simulink model "Rotor_and_Motor"  (R2022b)
settings: Solver=VariableStepAuto  StartTime=0.0  StopTime=20  MaxStep=.0001  RelTol=1e-3
InitFcn:
  | dir = pwd; %model directory
  | 
  | %go to look up tables
  | cd('..\Look Up Tables') %look up table directory
  | 
  | %Ct, Cp, and theta of rotor
  | load("Look Up Tables\BEMTdata_coax_final.mat");
  | 
  | %Peters-He model parameters (M,L,shape)
  | load("Look Up Tables\PetersHe_1state.mat");
  | 
  | %go back to model directory
  | cd(pwd);
  | 
  | %Ct, Cp, and theta of rotor
  | load("Look Up Tables\BEMTdata_coax_final.mat");
  | 
  | %Peters-He model parameters (M,L,shape)
  | load("Look Up Tables\PetersHe_1state.mat");
  | 
  | %rotor parameters
  | d_prop = 2*1.016;
  | R_c = d_prop/2*.12;
  | Nb = 2;
  | dr = rotor_params.dr;
  | Inertia = rotor_params.I_rotor;
  | kappa = rotor_params.kappa;
  | Cp0 = 5.908e-5;
  | 
  | %atmospheric properties
  | rho_air = 1.225;
  | 
  | 
  | %transmission properties
  | GR = 1.2;
  | wn = 101.0346; %transmission natural freq (rad/s)
  | zeta = 0.0106; %transmission damping ratio (-)
  | % wn = 30; %transmission natural freq (rad/s)
  | % zeta = 2*0.0106; %transmission damping ratio (-)
  | K = wn^2*Inertia; %belt stiffness
  | b = 2*zeta*sqrt(Inertia*K);%0.7706; %belt damping
  | % b = 1;
  | 
  | %model conditions
  | RPM0 = 945*GR;
  | RPMf = 975*GR;
  | ramp = 200*GR; %[rpm/s]
  | k = 0.865; %mass flow correction
  | shape = model.psi_a(1);
values from neighbouring files (symbols this model uses):
  Cp = [0.000195201118563 0.000195344815163 0.000195970524669 0.000196911243155 0.000198292722473 0.000199793715635 0.000201836164013 0.000204359459521 0.00020706119236 0.00020992934584 0.000212955219574 0.000216131124695 ... (150 elements, 1x150)]    [BEMT-1.mat]    (also in BEMT-2.mat = [5.908e-05 5.908e-05 5.908e-05 5.908e-05 5.908e-05 5.908e-05; BEMT-3.mat = [6.167e-05 6.167e-05 6.167e-05 6.167e-05 6.167e-05 6.1671725; BEMT-PF-Isolated-1.mat = [6.88284627296e-05 6.76929537705e-05 6.92283244838e-05 7.518; BEMT-PF-Isolated-2.mat = [6.88286203447e-05 6.76929720507e-05 6.92293837373e-05 7.518)
  Ct = [0 8.42066058624e-05 0.000168413211725 0.000252619817587 0.000348569118235 0.000435711397794 0.000522853677352 0.000609995956911 0.00069713823647 0.000784280516029 0.000871422795587 0.000958565075146 ... (150 elements, 1x150)]    [BEMT-1.mat]    (also in BEMT-2.mat = [-0.000241284312952 -0.00019885713846 -0.000156429963968 -0.; BEMT-3.mat = [-0.000252881464423 -0.00020500571035 -0.00015767832519 -0.0; BEMT-PF-Isolated-1.mat = [-0.000124730397385 6.78902114512e-07 0.000152796242494 0.00; BEMT-PF-Isolated-2.mat = [-0.000124743531158 6.68801957239e-07 0.000152879013625 0.00)
  model =     [DynInflow-1.mat]    (also in PP-1.mat; PP-2.mat; PP-3.mat)
  rotor_params =     [DynInflow-1.mat]    (also in PP-1.mat; PP-2.mat; PP-3.mat)
  theta = [-1.24244156171 -0.730247869575 -0.489791195362 -0.291308360013 -0.0904887039498 0.0775201787218 0.236938510902 0.389966557012 0.537998944025 0.680941129328 0.820002111662 0.955737387113 ... (150 elements, 1x150)]    [BEMT-1.mat]    (also in BEMT-2.mat = [-2.67472972391 -2.52181622329 -2.35655527709 -2.17339529035; BEMT-3.mat = [-2.61565298703 -2.45920727031 -2.29202818901 -2.11251263407; BEMT-PF-Isolated-1.mat = [-2 -1 0 1 2 3 4 5 6 7 8 9 ... (16 elements, 1x16)]; BEMT-PF-Isolated-2.mat = [-2 -1 0 1 2 3 4 5 6 7 8 9 ... (16 elements, 1x16)])
libraries: simulink x1
settings Model: PacingRate=0.010000  Creator=msa2925  LastModifiedBy=asper101

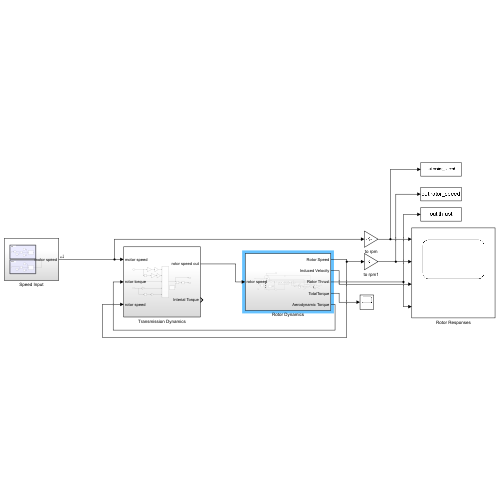
[thumbnail: Simulink's stored preview of the top-level diagram]
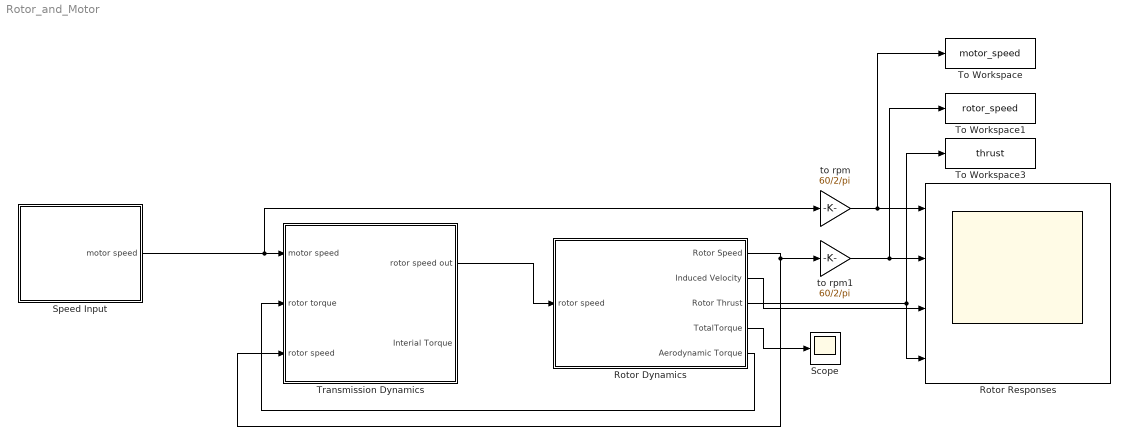
== system Rotor_and_Motor ==
  Rotor Dynamics : Subsystem
  Rotor Responses : Scope  NumInputPorts=4
  Scope : Scope
  Speed Input : Subsystem
  To Workspace : ToWorkspace  VariableName=motor_speed  SaveFormat=Timeseries  SampleTime=-1
  To Workspace1 : ToWorkspace  VariableName=rotor_speed  SaveFormat=Timeseries  SampleTime=-1
  To Workspace3 : ToWorkspace  VariableName=thrust  SaveFormat=Timeseries  SampleTime=-1
  Transmission Dynamics : Subsystem
  to rpm : Gain  Gain=60/2/pi
  to rpm1 : Gain  Gain=60/2/pi
  wires:
  Rotor Dynamics/1(Rotor Speed) -> Transmission Dynamics/3(rotor speed), to rpm1/1
  Rotor Dynamics/2(Induced Velocity) -> Rotor Responses/3
  Rotor Dynamics/3(Rotor Thrust) -> Rotor Responses/4, To Workspace3/1
  Rotor Dynamics/5(Aerodynamic Torque) -> Transmission Dynamics/2(rotor torque)
  Speed Input/1(motor speed) -> to rpm/1, Transmission Dynamics/1(motor speed)
  to rpm1/1 -> To Workspace1/1, Rotor Responses/2
  to rpm/1 -> To Workspace/1, Rotor Responses/1
  Rotor Dynamics/4(TotalTorque) -> Scope/1
  Transmission Dynamics/1(rotor speed out) -> Rotor Dynamics/1(rotor speed)

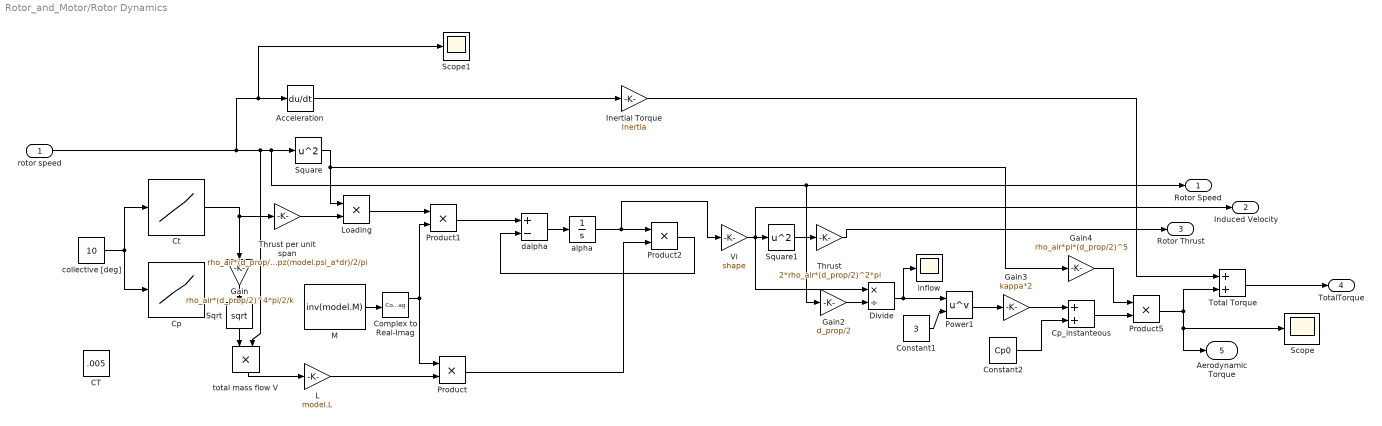
== system Rotor_and_Motor/Rotor Dynamics ==
  rotor speed : Inport
  Acceleration : Derivative
  CT : Constant  Value=.005
  Complex to Real-Imag : ComplexToRealImag
  Constant1 : Constant  Value=3
  Constant2 : Constant  Value=Cp0
  Cp : Lookup_n-D  NumberOfTableDimensions=1  BreakpointsForDimension1=theta  BreakpointsForDimension2=[1:3]  Table=Cp  InternalRulePriority=Speed  RndMeth=Simplest
  Cp_instanteous : Sum
  Ct : Lookup_n-D  NumberOfTableDimensions=1  BreakpointsForDimension1=theta  BreakpointsForDimension2=[1:3]  Table=Ct  InternalRulePriority=Speed  RndMeth=Simplest
  Divide : Product  Inputs=*/
  Gain : Gain  Gain=rho_air*(d_prop/2)^4*pi/2/k
  Gain2 : Gain  Gain=d_prop/2
  Gain3 : Gain  Gain=kappa*2
  Gain4 : Gain  Gain=rho_air*pi*(d_prop/2)^5
  Inertial Torque : Gain  Gain=Inertia
  L : Gain  Gain=model.L
  Loading : Product
  M : Constant  Value=inv(model.M)
  Power1 : Math  Operator=pow
  Product{,1..2,5} (4 alike) : Product
  Scope : Scope
  Scope1 : Scope
  Sqrt : Sqrt
  Square : Math  Operator=square
  Square1 : Math  Operator=square
  Thrust : Gain  Gain=2*rho_air*(d_prop/2)^2*pi
  Thrust per unit span : Gain  Gain=rho_air*(d_prop/2)^4*pi/(d_prop/2)*trapz(model.psi_a*dr)/2/pi
  Total Torque : Sum
  Vi : Gain  Gain=shape
  alpha : Integrator
  collective [deg] : Constant  Value=10
  dalpha : Sum  Inputs=+-
  inflow : Scope
  total mass flow V : Product
  Rotor Speed : Outport
  Induced Velocity : Outport  Port=2
  Rotor Thrust : Outport  Port=3
  TotalTorque : Outport  Port=4
  Aerodynamic Torque : Outport  Port=5
  wires:
  Gain/1 -> Sqrt/1
  L/1 -> Product/2
  total mass flow V/1 -> L/1
  collective [deg]/1 -> Cp/1, Ct/1
  Product2/1 -> dalpha/2
  rotor speed/1 -> Scope1/1, Acceleration/1, Square/1, Rotor Speed/1, Gain2/1, total mass flow V/2
  Vi/1 -> Induced Velocity/1, Divide/1, Square1/1
  Sqrt/1 -> total mass flow V/1
  Loading/1 -> Product1/1
  Product/1 -> Product2/2
  Square1/1 -> Thrust/1
  dalpha/1 -> alpha/1
  Thrust/1 -> Rotor Thrust/1
  Ct/1 -> Thrust per unit span/1, Gain/1
  M/1 -> Complex to Real-Imag/1
  Product1/1 -> dalpha/1
  alpha/1 -> Vi/1, Product2/1
  Complex to Real-Imag/1 -> Product1/2, Product/1
  Thrust per unit span/1 -> Loading/2
  Total Torque/1 -> TotalTorque/1
  Inertial Torque/1 -> Total Torque/1
  Acceleration/1 -> Inertial Torque/1
  Gain2/1 -> Divide/2
  Power1/1 -> Gain3/1
  Gain3/1 -> Cp_instanteous/1
  Constant2/1 -> Cp_instanteous/2
  Square/1 -> Loading/1, Gain4/1
  Gain4/1 -> Product5/1
  Cp_instanteous/1 -> Product5/2
  Constant1/1 -> Power1/2
  Divide/1 -> inflow/1, Power1/1
  Product5/1 -> Total Torque/2, Aerodynamic Torque/1, Scope/1

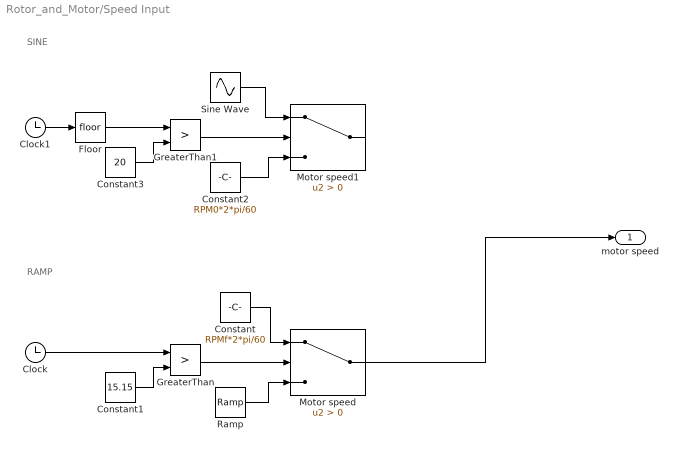
== system Rotor_and_Motor/Speed Input ==
  note: RAMP
  note: SINE
  Clock : Clock
  Clock1 : Clock
  Constant : Constant  Value=RPMf*2*pi/60
  Constant1 : Constant  Value=15.15
  Constant2 : Constant  Value=RPM0*2*pi/60
  Constant3 : Constant  Value=20
  Floor : Rounding
  GreaterThan : RelationalOperator  Operator=>  OutDataTypeStr=boolean  RndMeth=Simplest  InputSameDT=off
  GreaterThan1 : RelationalOperator  Operator=>  OutDataTypeStr=boolean  RndMeth=Simplest  InputSameDT=off
  Motor speed : Switch  Criteria=u2 > Threshold  SaturateOnIntegerOverflow=off  InputSameDT=off
  Motor speed1 : Switch  Criteria=u2 > Threshold  SaturateOnIntegerOverflow=off  InputSameDT=off
  Ramp : simulink/Sources/Ramp  slope=ramp*2*pi/60  start=15  InitialOutput=RPM0*2*pi/60
  Sine Wave : Sin  Amplitude=30*2*pi/60  Bias=RPM0*2*pi/60  Frequency=1*2*pi  SampleTime=0
  motor speed : Outport
  wires:
  GreaterThan/1 -> Motor speed/2
  Clock/1 -> GreaterThan/1
  Constant1/1 -> GreaterThan/2
  Ramp/1 -> Motor speed/3
  Constant/1 -> Motor speed/1
  GreaterThan1/1 -> Motor speed1/2
  Constant2/1 -> Motor speed1/3
  Constant3/1 -> GreaterThan1/2
  Clock1/1 -> Floor/1
  Sine Wave/1 -> Motor speed1/1
  Floor/1 -> GreaterThan1/1
  Motor speed/1 -> motor speed/1

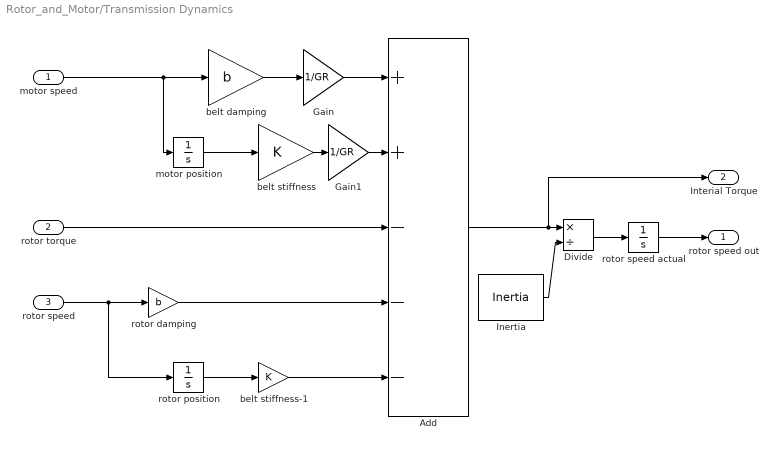
== system Rotor_and_Motor/Transmission Dynamics ==
  motor speed : Inport
  rotor torque : Inport  Port=2
  rotor speed : Inport  Port=3
  Add : Sum  Inputs=++---
  Divide : Product  Inputs=*/
  Gain : Gain  Gain=1/GR
  Gain1 : Gain  Gain=1/GR
  Inertia : Constant  Value=Inertia
  belt damping : Gain  Gain=b
  belt stiffness : Gain  Gain=K
  belt stiffness-1 : Gain  Gain=K
  motor position : Integrator
  rotor damping : Gain  Gain=b
  rotor position : Integrator
  rotor speed actual : Integrator  InitialCondition=RPM0/GR
  rotor speed out : Outport
  Interial Torque : Outport  Port=2
  wires:
  motor speed/1 -> belt damping/1, motor position/1
  motor position/1 -> belt stiffness/1
  rotor torque/1 -> Add/3
  rotor speed/1 -> rotor damping/1, rotor position/1
  belt stiffness-1/1 -> Add/5
  Add/1 -> Interial Torque/1, Divide/1
  Inertia/1 -> Divide/2
  Divide/1 -> rotor speed actual/1
  rotor speed actual/1 -> rotor speed out/1
  rotor position/1 -> belt stiffness-1/1
  belt stiffness/1 -> Gain1/1
  Gain1/1 -> Add/2
  belt damping/1 -> Gain/1
  Gain/1 -> Add/1
  rotor damping/1 -> Add/4
